simulink model "biorreactorinterfaz"  (R2017a)
settings: Solver=ode45  StartTime=0.0  StopTime=inf  MaxStep=3000  RelTol=1e-3  EnableMultiTasking=on
undefined symbols (not defined in the file): printf
libraries: instrumentlib x2
settings Model: Creator=julian  LastModifiedBy=jncre
settings DataIOCC: LimitDataPoints=on  SaveFormat=Array
settings OptimizationCC: LifeSpan=inf
settings DebuggingCC: SolverPrmCheckMsg=warning  SFUnexpectedBacktrackingDiag=warning  SFNoUnconditionalDefaultTransitionDiag=warning  SFExecutionAtInitializationDiag=none
settings HardwareCC: ProdBitPerPointer=32  ProdBitPerSizeT=32  ProdBitPerPtrDiffT=32  ProdLargestAtomicFloat=None  ProdIntDivRoundTo=Undefined  ProdEndianess=Unspecified  ProdWordSize=32  ProdHWDeviceType=32-bit Generic
settings ModelReferenceCC: PropagateSignalLabelsOutOfModel=off
settings GRTTargetCC: TargetLangStandard=C89/C90 (ANSI)  GeneratePreprocessorConditionals=Disable all
settings ConfigComp: CovMetricSettings=dw  CovHtmlReporting=on  CovSaveCumulativeToWorkspaceVar=on  CovSaveSingleToWorkspaceVar=on  CovExternalEMLEnable=off  CovSFcnEnable=off

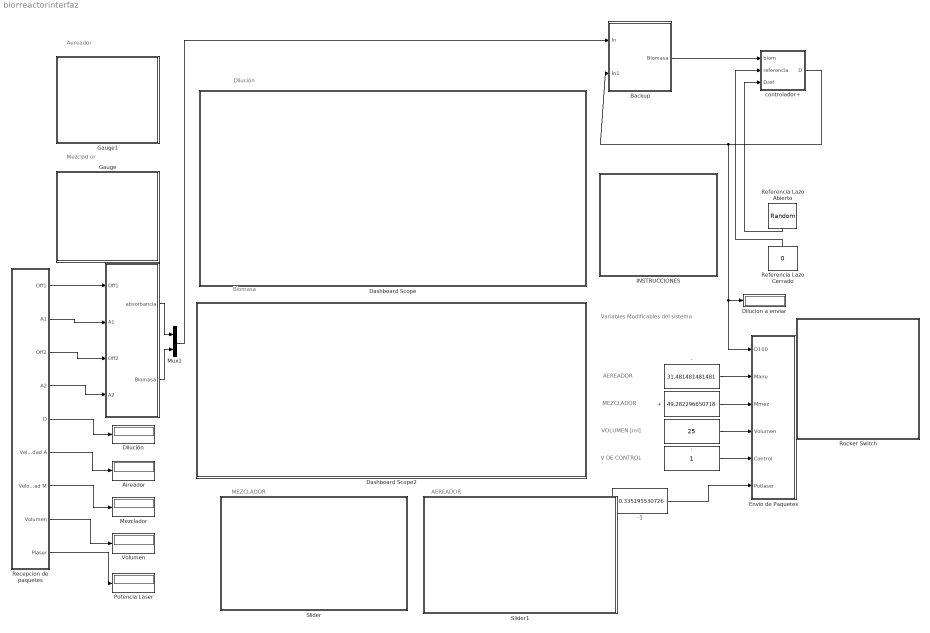
== system biorreactorinterfaz ==
  note: MEZCLADOR
  note: Variables Modificables del sistema
  note: Aereador
  note: Mezclad or
  note: Dilución
  note: Biomasa
  note: AEREADOR
  note: VOLUMEN [ml]
  note: V DE CONTROL
  note: MEZCLADOR
  note: AEREADOR
  " " : Subsystem
  "    " : Constant  OutMin=[0]  OutMax=[255]
  "  Referencia Lazo Abierto" : RandomNumber  Variance=0  SampleTime=60
  "  Referencia Lazo Cerrado" : Constant  Value=0  OutMin=[0]  OutMax=[255]
  + : Constant  Value=49.282296650718  OutMin=[0]  OutMax=[255]
  - : Constant  Value=31.481481481481  OutMin=[0]  OutMax=[255]
  -1 : Constant  Value=10.335195530726  OutMin=[0]  OutMax=[255]
  . : Constant  Value=25  OutMin=[0]  OutMax=[255]
  Aireador : Display
  "Backup " : Subsystem
  Dashboard Scope : Subsystem  DialogController=hmiCreateDDGDialog  IsWebBlock=on  mask(MWDashboardBlock){webBlockId=8c9dad69-430c-4d74-ad86-4bac776ac25d, webBlockType=sdiscope, ShowInitialText=on, HMISrcModelName=biorreactorinterfaz}
      mask prompts: webBlockId "WebBlock Id"; webBlockType "WebBlock Type"; HMISrcModelName "Source Model"
      mask help: SimulinkHMI:dialogs:HMIScopeDialogDesc
      mask Help: helpview([docroot '/mapfiles/simulink.map'], 'hmi_scope')
      mask Display:
      | if strcmp(get_param(bdroot(gcb),'BlockDiagramType'), 'library')
      |     image([(matlabroot) '/toolbox/simulink/hmi/icons/DashboardScope.png']);
      | end
  Dashboard Scope2 : Subsystem  DialogController=hmiCreateDDGDialog  IsWebBlock=on  mask(MWDashboardBlock){webBlockId=8b4aa089-d446-4a71-ab19-24e3a6b59003, webBlockType=sdiscope, ShowInitialText=on, HMISrcModelName=biorreactorinterfaz}
      mask prompts: webBlockId "WebBlock Id"; webBlockType "WebBlock Type"; HMISrcModelName "Source Model"
      mask help: SimulinkHMI:dialogs:HMIScopeDialogDesc
      mask Help: helpview([docroot '/mapfiles/simulink.map'], 'hmi_scope')
      mask Display:
      | if strcmp(get_param(bdroot(gcb),'BlockDiagramType'), 'library')
      |     image([(matlabroot) '/toolbox/simulink/hmi/icons/DashboardScope.png']);
      | end
  "Dilucion a enviar " : Display
  "Dilución " : Display
  "Envio de Paquetes " : Subsystem
  Gauge : Subsystem  DialogController=hmiCreateDDGDialog  IsWebBlock=on  mask(MWDashboardBlock){webBlockId=1771e7b1-d5a9-4a2a-b403-68d7d56c6e4f, webBlockType=circulargauge, ShowInLibBrowser=on, ShowInitialText=on, HMISrcModelName=biorreactorinterfaz}
      mask prompts: webBlockId "WebBlock Id"; webBlockType "WebBlock Type"; HMISrcModelName "Source Model"
      mask help: SimulinkHMI:dialogs:CircularGaugeDialogDesc
      mask Help: helpview([docroot '/mapfiles/simulink.map'], 'hmi_gauge')
      mask Display:
      | if strcmp(get_param(bdroot(gcb),'BlockDiagramType'), 'library')
      |     image([(matlabroot) '/toolbox/simulink/hmi/icons/CircularGauge.png']);
      | end
  Gauge1 : Subsystem  DialogController=hmiCreateDDGDialog  IsWebBlock=on  mask(MWDashboardBlock){webBlockId=77ca28d1-152a-4355-9c8a-97edce774be2, webBlockType=circulargauge, ShowInLibBrowser=on, ShowInitialText=on, HMISrcModelName=biorreactorinterfaz}
      mask prompts: webBlockId "WebBlock Id"; webBlockType "WebBlock Type"; HMISrcModelName "Source Model"
      mask help: SimulinkHMI:dialogs:CircularGaugeDialogDesc
      mask Help: helpview([docroot '/mapfiles/simulink.map'], 'hmi_gauge')
      mask Display:
      | if strcmp(get_param(bdroot(gcb),'BlockDiagramType'), 'library')
      |     image([(matlabroot) '/toolbox/simulink/hmi/icons/CircularGauge.png']);
      | end
  "INSTRUCCIONES " : Subsystem
      mask Display: image('C:\Users\Plantas\Desktop\imagenes\manual-154693_960_720.png');
  Mezclador : Display
  Mux1 : Mux  Inputs=2
  Potencia Laser : Display
  Recepcion de paquetes : Subsystem
  Rocker Switch : Subsystem  DialogController=hmiCreateDDGDialog  IsWebBlock=on  mask(MWDashboardBlock){webBlockId=eba58b42-0445-4a4d-9247-ee86cb05d07f, webBlockType=rockerswitch, ShowInLibBrowser=on, ShowInitialText=on, HMISrcModelName=biorreactorinterfaz}
      mask prompts: webBlockId "WebBlock Id"; webBlockType "WebBlock Type"; HMISrcModelName "Source Model"
      mask help: SimulinkHMI:dialogs:SwitchDialogDesc
      mask Help: helpview([docroot '/mapfiles/simulink.map'], 'hmi_rocker_switch')
      mask Display:
      | if strcmp(get_param(bdroot(gcb),'BlockDiagramType'), 'library')
      |     image([(matlabroot) '/toolbox/simulink/hmi/icons/RockerSwitch.png']);
      | end
  Slider : Subsystem  DialogController=hmiCreateDDGDialog  IsWebBlock=on  mask(MWDashboardBlock){webBlockId=72a49820-ff40-447c-a531-f8c26b851cc1, webBlockType=slider, ShowInLibBrowser=on, ShowInitialText=on, HMISrcModelName=biorreactorinterfaz}
      mask prompts: webBlockId "WebBlock Id"; webBlockType "WebBlock Type"; HMISrcModelName "Source Model"
      mask help: SimulinkHMI:dialogs:SliderDialogDesc
      mask Help: helpview([docroot '/mapfiles/simulink.map'], 'hmi_slider')
      mask Display:
      | if strcmp(get_param(bdroot(gcb),'BlockDiagramType'), 'library')
      |     image([(matlabroot) '/toolbox/simulink/hmi/icons/Slider.png']);
      | end
  Slider1 : Subsystem  DialogController=hmiCreateDDGDialog  IsWebBlock=on  mask(MWDashboardBlock){webBlockId=74fe66a2-b3d6-4ef4-9024-48ee337486ba, webBlockType=slider, ShowInLibBrowser=on, ShowInitialText=on, HMISrcModelName=biorreactorinterfaz}
      mask prompts: webBlockId "WebBlock Id"; webBlockType "WebBlock Type"; HMISrcModelName "Source Model"
      mask help: SimulinkHMI:dialogs:SliderDialogDesc
      mask Help: helpview([docroot '/mapfiles/simulink.map'], 'hmi_slider')
      mask Display:
      | if strcmp(get_param(bdroot(gcb),'BlockDiagramType'), 'library')
      |     image([(matlabroot) '/toolbox/simulink/hmi/icons/Slider.png']);
      | end
  Volumen : Display
  controlador+ : Subsystem
  wires:
  ./1 -> "Envio de Paquetes "/4(Volumen)
  Recepcion de paquetes/6("Velocidad A ") -> Aireador/1
  Recepcion de paquetes/7(Velocidad M) -> Mezclador/1
  Recepcion de paquetes/5(D) -> "Dilución "/1
  "Backup "/1(Biomasa) -> controlador+/1(biom)
  Mux1/1 -> "Backup "/1(In)
  " "/1(absorbancia) -> Mux1/1
  " "/2("Biomasa ") -> Mux1/2
  Recepcion de paquetes/8(Volumen) -> Volumen/1
  controlador+/1(D) -> "Envio de Paquetes "/1(D100), "Dilucion a enviar "/1, "Backup "/2(In1)
  "  Referencia Lazo Abierto"/1 -> controlador+/3(Dref)
  "  Referencia Lazo Cerrado"/1 -> controlador+/2(referencia)
  -/1 -> "Envio de Paquetes "/2(Maire)
  +/1 -> "Envio de Paquetes "/3(Mmez)
  "    "/1 -> "Envio de Paquetes "/5(Control)
  -1/1 -> "Envio de Paquetes "/6(Potlaser)
  Recepcion de paquetes/9(Plaser) -> Potencia Laser/1
  Recepcion de paquetes/2("A1 ") -> " "/2(A1)
  Recepcion de paquetes/1(Off1) -> " "/1(Off1)
  Recepcion de paquetes/3(Off2) -> " "/3(Off2)
  Recepcion de paquetes/4("A2 ") -> " "/4(A2)

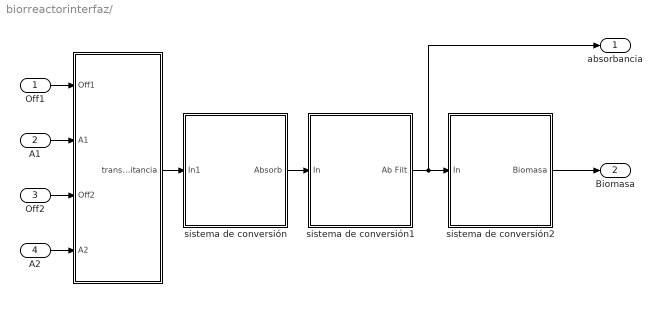
== system biorreactorinterfaz/  ==
  Off1 : Inport
  A1 : Inport  Port=2
  Off2 : Inport  Port=3
  A2 : Inport  Port=4
  " " : Subsystem
  sistema de conversión : Subsystem
  sistema de conversión1 : Subsystem
  sistema de conversión2 : Subsystem
  absorbancia : Outport
  "Biomasa " : Outport  Port=2
  wires:
  sistema de conversión2/1(Biomasa) -> "Biomasa "/1
  A1/1 -> " "/2(A1)
  " "/1("transmitancia ") -> sistema de conversión/1(In1)
  sistema de conversión/1(Absorb) -> sistema de conversión1/1(In)
  Off2/1 -> " "/3(Off2)
  sistema de conversión1/1(Ab Filt) -> absorbancia/1, sistema de conversión2/1(In)
  Off1/1 -> " "/1(Off1)
  A2/1 -> " "/4(A2)

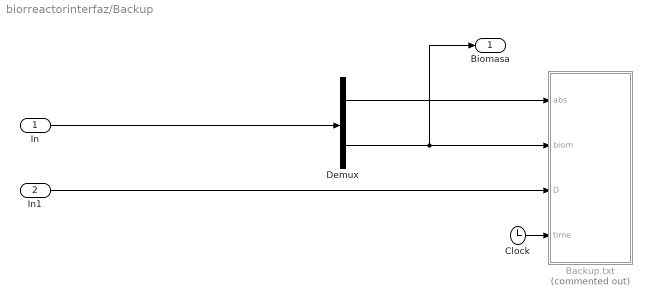
== system biorreactorinterfaz/Backup  ==
  In : Inport
  In1 : Inport  Port=2
  Backup.txt : MATLAB Function  Commented=on  TreatAsAtomicUnit=on
  Clock : Clock
  Demux : Demux  Outputs=2
  Biomasa : Outport
  wires:
  Clock/1 -> Backup.txt/4(time)
  In1/1 -> Backup.txt/3(D)
  Demux/2 -> Biomasa/1, Backup.txt/2(biom)
  Demux/1 -> Backup.txt/1(abs)
  In/1 -> Demux/1

== system biorreactorinterfaz/Dashboard Scope ==

== system biorreactorinterfaz/Dashboard Scope2 ==

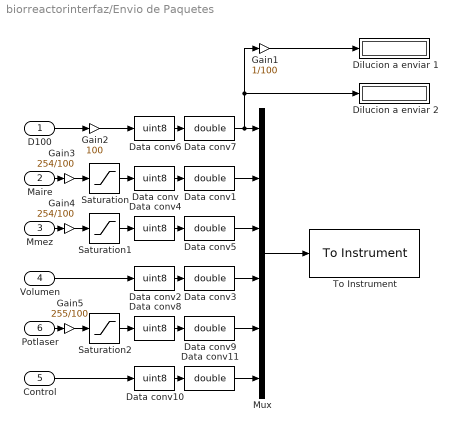
== system biorreactorinterfaz/Envio de Paquetes  ==
  D100 : Inport
  Maire : Inport  Port=2
  Mmez : Inport  Port=3
  Volumen : Inport  Port=4
  Control : Inport  Port=5
  Potlaser : Inport  Port=6
  Data conv{,2,4,6,8,10} (6 alike) : DataTypeConversion  OutDataTypeStr=uint8
  Data conv{1,3,5,7,9,11} (6 alike) : DataTypeConversion  OutDataTypeStr=double
  Dilucion a enviar 1 : Display
  Dilucion a enviar 2 : Display
  Gain1 : Gain  Gain=1/100
  Gain2 : Gain  Gain=100
  Gain3 : Gain  Gain=254/100
  Gain4 : Gain  Gain=254/100
  Gain5 : Gain  Gain=255/100
  Mux : Mux  Inputs=6
  Saturation : Saturate  UpperLimit=254  LowerLimit=0
  Saturation1 : Saturate  UpperLimit=254  LowerLimit=0
  Saturation2 : Saturate  UpperLimit=255  LowerLimit=0
  To Instrument : instrumentlib/To Instrument  sampleTime=60  isWorkspaceObject=off  timeout=30000  inputBufferSize=200  protocol=Serial  serialPort=COM4  baudRate=9600  gpibVendor=Agilent Technologies  boardIndex=0  primaryAddress=1  secondaryAddress=0  visaVendor=Agilent  visaSerialPort=0  chassisIndex=0  logicalAddress=0  tcpRemoteHost='127.0.0.1'  tcpRemotePort=4500  udpRemoteHost='127.0.0.1'  udpRemotePort=9090  visaTCPBoardIndex=0  visaTCPRemoteHost='127.0.0.1'  usbBoardIndex=0  usbManufID=0  usbModelCode=0  usbSerialNumber=0  initAction=None  initCommand='G 0 70 100 0 255 1 F\n'  initFunction="printf(\"INICIO:0.1 125 5/n\")"  command=''  sendFormat=ASCII  asciiFormatting='G %i %i %i %i %i %i F\n'  precision=32-bit integer  byteOrder=Little endian
      settings: SourceProductName=Instrument Control Toolbox  SourceProductBaseCode=IC
  wires:
  Mmez/1 -> Gain4/1
  Volumen/1 -> Data conv2/1
  Mux/1 -> To Instrument/1
  Data conv/1 -> Data conv1/1
  Data conv1/1 -> Mux/2
  Gain1/1 -> Dilucion a enviar 1/1
  Data conv2/1 -> Data conv3/1
  Data conv3/1 -> Mux/4
  Data conv4/1 -> Data conv5/1
  Data conv5/1 -> Mux/3
  Data conv6/1 -> Data conv7/1
  Data conv7/1 -> Dilucion a enviar 2/1, Gain1/1, Mux/1
  Data conv9/1 -> Mux/5
  Data conv8/1 -> Data conv9/1
  Data conv10/1 -> Data conv11/1
  Control/1 -> Data conv10/1
  Data conv11/1 -> Mux/6
  D100/1 -> Gain2/1
  Gain2/1 -> Data conv6/1
  Saturation1/1 -> Data conv4/1
  Gain3/1 -> Saturation/1
  Saturation/1 -> Data conv/1
  Gain4/1 -> Saturation1/1
  Maire/1 -> Gain3/1
  Gain5/1 -> Saturation2/1
  Potlaser/1 -> Gain5/1
  Saturation2/1 -> Data conv8/1

== system biorreactorinterfaz/Gauge ==

== system biorreactorinterfaz/Gauge1 ==

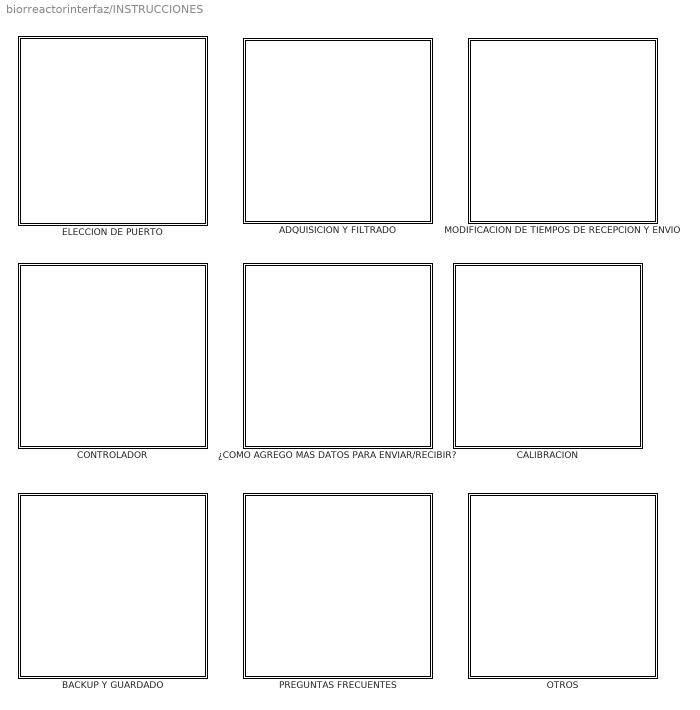
== system biorreactorinterfaz/INSTRUCCIONES  ==
  "ADQUISICION Y FILTRADO " : Subsystem
  BACKUP Y GUARDADO : Subsystem
  CALIBRACION : Subsystem
  CONTROLADOR : Subsystem
  "ELECCION DE PUERTO " : Subsystem
  MODIFICACION DE TIEMPOS DE RECEPCION Y ENVIO : Subsystem
  "OTROS " : Subsystem
  PREGUNTAS FRECUENTES : Subsystem
  ¿COMO AGREGO MAS DATOS PARA ENVIAR/RECIBIR? : Subsystem

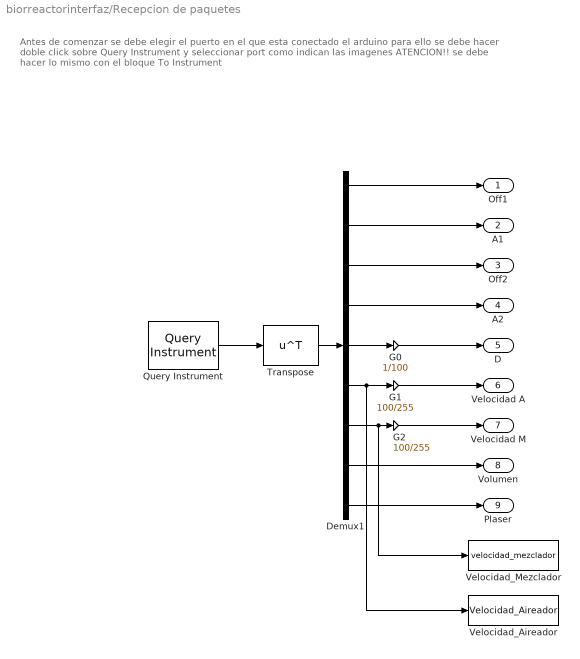
== system biorreactorinterfaz/Recepcion de paquetes ==
  note: Antes de comenzar se debe elegir el puerto en el que esta conectado el arduino
      | para ello se debe hacer doble click sobre Query Instrument y seleccionar port
      | como indican las imagenes
      | ATENCION!! se debe hacer lo mismo con el bloque To Instrument
  Demux1 : Demux  Outputs=9
  G0 : Gain  Gain=1/100
  G1 : Gain  Gain=100/255
  G2 : Gain  Gain=100/255
  Query Instrument : instrumentlib/Query Instrument  sampleTime=3  isWorkspaceObject=off  timeout=90  inputBufferSize=1200  protocol=Serial  serialPort=COM4  baudRate=9600  gpibVendor=Agilent Technologies  boardIndex=0  primaryAddress=1  secondaryAddress=0  visaVendor=Agilent  visaSerialPort=0  chassisIndex=0  logicalAddress=0  tcpRemoteHost='127.0.0.1'  tcpRemotePort=4500  udpRemoteHost='127.0.0.1'  udpRemotePort=9090  visaTCPBoardIndex=0  visaTCPRemoteHost='127.0.0.1'  usbBoardIndex=0  usbManufID=0  usbModelCode=0  usbSerialNumber=0  initAction=Send ASCII Commands  initCommand='G 0 70 100 0 255 1 F\n'  initFunction=get  queryCommand=''  responseFormat=ASCII  asciiFormatting='S,%d,%d,%d,%d,%d,%d,%d,%d,%d,E'  precision=8-bit integer  byteOrder=Little endian  valuesToRead=1  removeBytes=on  afterOutputAction=Repeat query for new data  enableFrames=on  frameSize=9
      settings: SourceProductName=Instrument Control Toolbox  SourceProductBaseCode=IC
  Transpose : Math  Operator=transpose  SaturateOnIntegerOverflow=on
  Velocidad_Aireador : ToWorkspace  VariableName=Velocidad_Aireador  SaveFormat=Timeseries  SampleTime=-1
      settings: Save2DSignal=2-D array (concatenate along first dimension)
  Velocidad_Mezclador : ToWorkspace  VariableName=velocidad_mezclador  SaveFormat=Timeseries  SampleTime=-1
      settings: Save2DSignal=2-D array (concatenate along first dimension)
  Off1 : Outport
  "A1 " : Outport  Port=2
  Off2 : Outport  Port=3
  "A2 " : Outport  Port=4
  D : Outport  Port=5
  "Velocidad A " : Outport  Port=6
  Velocidad M : Outport  Port=7
  Volumen : Outport  Port=8
  Plaser : Outport  Port=9
  wires:
  Demux1/4 -> "A2 "/1
  Demux1/5 -> G0/1
  Demux1/7 -> Velocidad_Mezclador/1, G2/1
  Transpose/1 -> Demux1/1
  Query Instrument/1 -> Transpose/1
  Demux1/6 -> Velocidad_Aireador/1, G1/1
  Demux1/1 -> Off1/1
  G2/1 -> Velocidad M/1
  G1/1 -> "Velocidad A "/1
  G0/1 -> D/1
  Demux1/8 -> Volumen/1
  Demux1/9 -> Plaser/1
  Demux1/2 -> "A1 "/1
  Demux1/3 -> Off2/1

== system biorreactorinterfaz/Rocker Switch ==

== system biorreactorinterfaz/Slider ==

== system biorreactorinterfaz/Slider1 ==

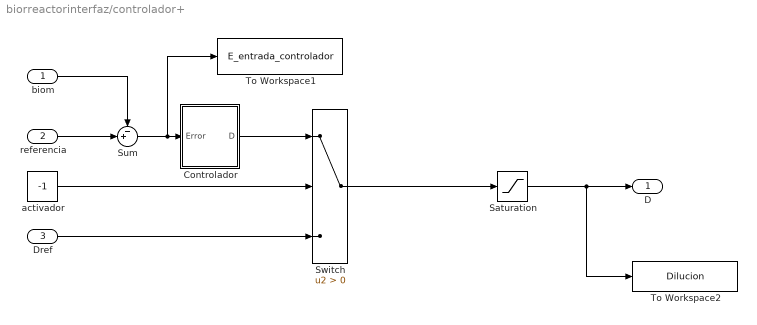
== system biorreactorinterfaz/controlador+ ==
  biom : Inport
  referencia : Inport  Port=2
  Dref : Inport  Port=3
  Controlador : Subsystem
  Saturation : Saturate  UpperLimit=1  LowerLimit=0
  Sum : Sum  Inputs=-+|
  Switch : Switch  Criteria=u2 > Threshold
  To Workspace1 : ToWorkspace  VariableName=E_entrada_controlador  SaveFormat=Timeseries  SampleTime=-1
      settings: Save2DSignal=2-D array (concatenate along first dimension)
  To Workspace2 : ToWorkspace  VariableName=Dilucion  SaveFormat=Timeseries  SampleTime=-1
      settings: Save2DSignal=2-D array (concatenate along first dimension)
  activador : Constant  Value=-1
  D : Outport
  wires:
  activador/1 -> Switch/2
  Dref/1 -> Switch/3
  Switch/1 -> Saturation/1
  Sum/1 -> To Workspace1/1, Controlador/1(Error)
  biom/1 -> Sum/1
  referencia/1 -> Sum/2
  Controlador/1(D) -> Switch/1
  Saturation/1 -> To Workspace2/1, D/1

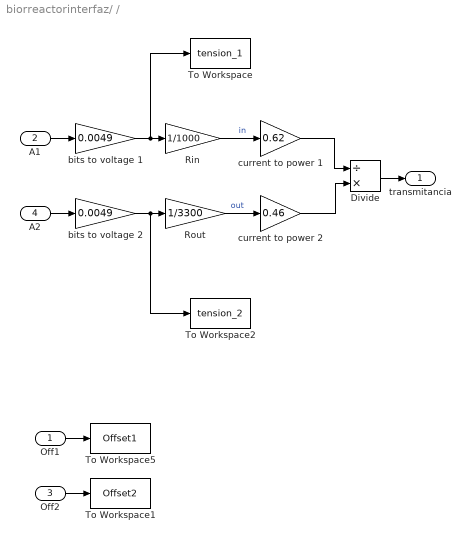
== system biorreactorinterfaz/ /  ==
  Off1 : Inport
  A1 : Inport  Port=2
  Off2 : Inport  Port=3
  A2 : Inport  Port=4
  Divide : Product  Inputs=/*
  Rin : Gain  Gain=1/1000
  "Rout " : Gain  Gain=1/3300
  To Workspace : ToWorkspace  VariableName=tension_1  SaveFormat=Timeseries  SampleTime=-1
  To Workspace1 : ToWorkspace  VariableName=Offset2  SaveFormat=Timeseries  SampleTime=-1
  To Workspace2 : ToWorkspace  VariableName=tension_2  SaveFormat=Timeseries  SampleTime=-1
  To Workspace5 : ToWorkspace  VariableName=Offset1  SaveFormat=Timeseries  SampleTime=-1
  "bits to voltage 1 " : Gain  Gain=0.0049
  bits to voltage 2 : Gain  Gain=0.0049
  current to power 1 : Gain  Gain=0.62
  current to power 2 : Gain  Gain=0.46
  "transmitancia " : Outport
  wires:
  "Rout "/1 -> current to power 2/1  "out"
  Rin/1 -> current to power 1/1  "in"
  "bits to voltage 1 "/1 -> To Workspace/1, Rin/1
  bits to voltage 2/1 -> To Workspace2/1, "Rout "/1
  current to power 2/1 -> Divide/2
  Divide/1 -> "transmitancia "/1
  A1/1 -> "bits to voltage 1 "/1
  A2/1 -> bits to voltage 2/1
  Off1/1 -> To Workspace5/1
  Off2/1 -> To Workspace1/1
  current to power 1/1 -> Divide/1

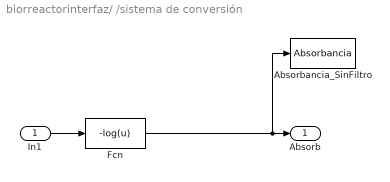
== system biorreactorinterfaz/ /sistema de conversión ==
  In1 : Inport
  Absorbancia_SinFiltro : ToWorkspace  VariableName=Absorbancia  SaveFormat=Timeseries  SampleTime=-1
      settings: Save2DSignal=2-D array (concatenate along first dimension)
  Fcn : Fcn  Expr=-log(u)
  Absorb : Outport
  wires:
  In1/1 -> Fcn/1
  Fcn/1 -> Absorbancia_SinFiltro/1, Absorb/1

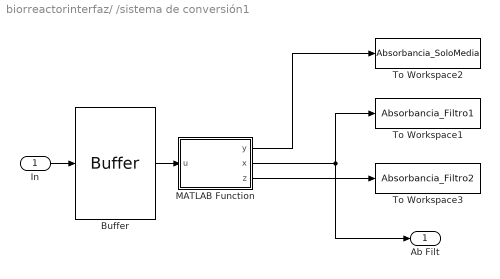
== system biorreactorinterfaz/ /sistema de conversión1 ==
  In : Inport
  Buffer : Buffer  N=20  OutputFrames=off
  MATLAB Function : MATLAB Function  TreatAsAtomicUnit=on
  To Workspace1 : ToWorkspace  VariableName=Absorbancia_Filtro1  SaveFormat=Timeseries  SampleTime=-1
      settings: Save2DSignal=2-D array (concatenate along first dimension)
  To Workspace2 : ToWorkspace  VariableName=Absorbancia_SoloMedia  SaveFormat=Timeseries  SampleTime=-1
      settings: Save2DSignal=2-D array (concatenate along first dimension)
  To Workspace3 : ToWorkspace  VariableName=Absorbancia_Filtro2  SaveFormat=Timeseries  SampleTime=-1
      settings: Save2DSignal=2-D array (concatenate along first dimension)
  Ab Filt : Outport
  wires:
  In/1 -> Buffer/1
  Buffer/1 -> MATLAB Function/1(u)
  MATLAB Function/2(x) -> Ab Filt/1, To Workspace1/1
  MATLAB Function/1(y) -> To Workspace2/1
  MATLAB Function/3(z) -> To Workspace3/1

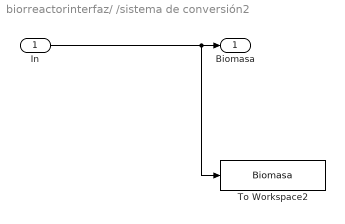
== system biorreactorinterfaz/ /sistema de conversión2 ==
  In : Inport
  To Workspace2 : ToWorkspace  VariableName=Biomasa  SaveFormat=Timeseries  SampleTime=-1
      settings: Save2DSignal=2-D array (concatenate along first dimension)
  Biomasa : Outport
  wires:
  In/1 -> To Workspace2/1, Biomasa/1

== system biorreactorinterfaz/INSTRUCCIONES /ADQUISICION Y FILTRADO  ==

== system biorreactorinterfaz/INSTRUCCIONES /BACKUP Y GUARDADO ==

== system biorreactorinterfaz/INSTRUCCIONES /CALIBRACION ==

== system biorreactorinterfaz/INSTRUCCIONES /CONTROLADOR ==

== system biorreactorinterfaz/INSTRUCCIONES /ELECCION DE PUERTO  ==
  note: *El bloque " Query Instrument" se encuentra adentro del subsistema "Recepcion de paquetes"
      | *El bloque "To Instrument" senencuentra en el subsistema "Envio de paquetes "
  note: Antes de comenzar se debe elegir el puerto en el que esta conectado el arduino
      | para ello se debe hacer doble click sobre Query Instrument y seleccionar port
      | como indican las imagenes
      | ATENCION!! se debe hacer lo mismo con el bloque To Instrument

== system biorreactorinterfaz/INSTRUCCIONES /MODIFICACION DE TIEMPOS DE RECEPCION Y ENVIO ==

== system biorreactorinterfaz/INSTRUCCIONES /OTROS  ==

== system biorreactorinterfaz/INSTRUCCIONES /PREGUNTAS FRECUENTES ==

== system biorreactorinterfaz/INSTRUCCIONES /¿COMO AGREGO MAS DATOS PARA ENVIAR//RECIBIR? ==

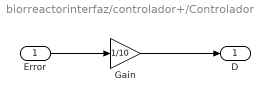
== system biorreactorinterfaz/controlador+/Controlador ==
  Error : Inport
  Gain : Gain  Gain=1/10
  D : Outport
  wires:
  Error/1 -> Gain/1
  Gain/1 -> D/1

== matlab function biorreactorinterfaz/Backup /Backup.txt ==
  data: abs input; biom input; D input; time input
function fcn(abs,biom,D,time)

fileID = fopen('backup.m','a+');

fprintf(fileID,'%l,%f,%f,%f\n',time,abs,D,biom);

fclose(fileID);

== matlab function biorreactorinterfaz/ /sistema de conversión1/MATLAB Function ==
  data: u input; y output; x output; z output
function [y,x,z]= fcn(u)
n= length(u);
x1= sort(u);

a= floor(n/4);
b= floor(3*n/4);

z1= x1(1:b);
x2= x1(a:b);


y= mean(u);
x= mean(x2);
z= mean(z1);
